simulink model "flc_ruido"  (R2023a)
settings: Solver=VariableStepAuto  StartTime=0.0  StopTime=1000  RelTol=1e-3
values from neighbouring files (symbols this model uses):
  A = 0.0154    [parametros.m]    (also in variables.mat)
  az1 = 1    [parametros.m]    (also in variables.mat)
  az2 = 1    [parametros.m]    (also in variables.mat)
  az3 = 1    [parametros.m]    (also in variables.mat)
  g = 9.8    [parametros.m]    (also in variables.mat)
  H_star1 = 0.4    [parametros.m]    (also in variables.mat)
  H_star2 = 0.15    [parametros.m]    (also in variables.mat)
  Sn = 5e-5    (= 5e-05)    [parametros.m]    (also in variables.mat)
libraries: fuzblock x2
settings Model: Creator=empg0  LastModifiedBy=empg0

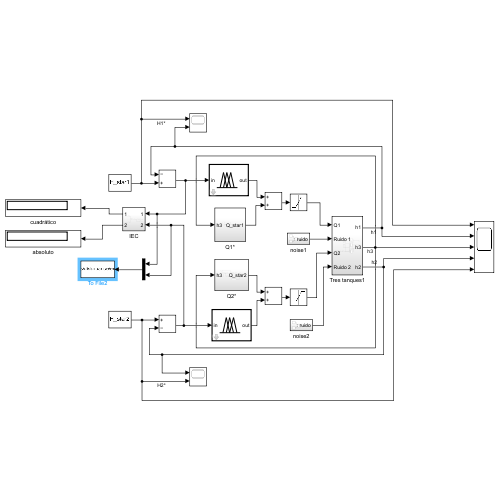
[thumbnail: Simulink's stored preview of the top-level diagram]
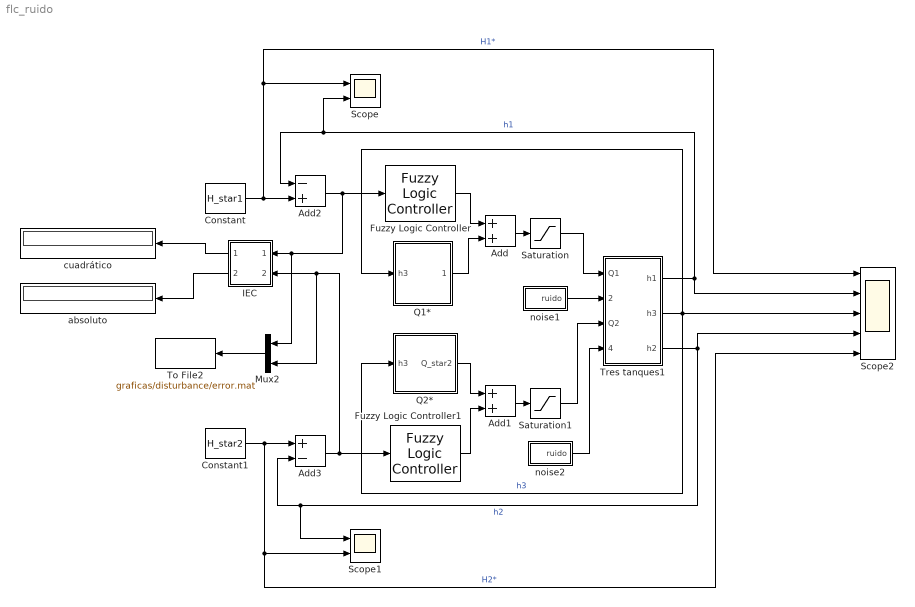
== system flc_ruido ==
  Add : Sum
  Add1 : Sum
  Add2 : Sum  Inputs=-+
  Add3 : Sum  Inputs=+-
  Constant : Constant  Value=H_star1
  Constant1 : Constant  Value=H_star2
  Fuzzy Logic Controller : fuzblock/Fuzzy Logic  Controller  FIS='error_fuzzy.fis'  OutputSampleNumber=101  DataType=double  FuzzifiedInputs=off  RuleFiringStrengths=off  RuleOutputs=off  AggregatedOutputs=off  SimulateUsing=Interpreted execution  OutOfRangeInputValueMessage=warning  NoRuleFiredMessage=warning  EmptyOutputFuzzySetMessage=warning
  Fuzzy Logic Controller1 : fuzblock/Fuzzy Logic  Controller  FIS='error_fuzzy.fis'  OutputSampleNumber=101  DataType=double  FuzzifiedInputs=off  RuleFiringStrengths=off  RuleOutputs=off  AggregatedOutputs=off  SimulateUsing=Interpreted execution  OutOfRangeInputValueMessage=warning  NoRuleFiredMessage=warning  EmptyOutputFuzzySetMessage=warning
  IEC : Subsystem
  Mux2 : Mux  Inputs=2
  Q1* : Subsystem
  Q2* : Subsystem
  Saturation : Saturate  UpperLimit=0.1  LowerLimit=0
  Saturation1 : Saturate  UpperLimit=0.1  LowerLimit=0
  Scope : Scope  NumInputPorts=2
  Scope1 : Scope  NumInputPorts=2
  Scope2 : Scope  NumInputPorts=5
  To File2 : ToFile  Filename=graficas/disturbance/error.mat  MatrixName=error  SampleTime=0.5
  Tres tanques1 : Subsystem
  absoluto : Display
  cuadrático : Display
  noise1 : Subsystem
  noise2 : Subsystem
  wires:
  Fuzzy Logic Controller/1 -> Add/1
  Q1*/1(Q_star1) -> Add/2
  Q2*/1(Q_star2) -> Add1/1
  Fuzzy Logic Controller1/1 -> Add1/2
  Constant/1 -> Scope/1, Scope2/1, Add2/2  "H1*"
  Add2/1 -> Mux2/1, IEC/1(In1), Fuzzy Logic Controller/1
  Tres tanques1/1(h1) -> Scope2/2, Scope/2, Add2/1  "h1"
  Add3/1 -> Mux2/2, IEC/2(In2), Fuzzy Logic Controller1/1
  Constant1/1 -> Scope1/2, Scope2/5, Add3/1  "H2*"
  Tres tanques1/3(h2) -> Scope2/4, Scope1/1, Add3/2  "h2"
  Tres tanques1/2(h3) -> Scope2/3, Q1*/1(h3), Q2*/1(h3)  "h3"
  Add/1 -> Saturation/1
  Add1/1 -> Saturation1/1
  IEC/1(Out1) -> cuadrático/1
  Mux2/1 -> To File2/1
  Saturation/1 -> Tres tanques1/1(Q1)
  Saturation1/1 -> Tres tanques1/3(Q2)
  noise1/1(ruido) -> Tres tanques1/2(Ruido 1)
  noise2/1(ruido) -> Tres tanques1/4(Ruido 2)
  IEC/2(Out2) -> absoluto/1

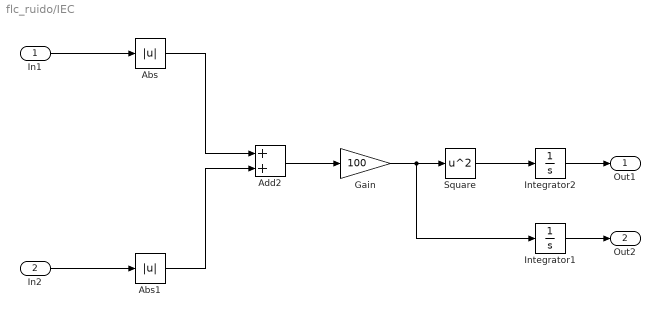
== system flc_ruido/IEC ==
  In1 : Inport
  In2 : Inport  Port=2
  Abs : Abs  SaturateOnIntegerOverflow=off
  Abs1 : Abs  SaturateOnIntegerOverflow=off
  Add2 : Sum
  Gain : Gain  Gain=100
  Integrator1 : Integrator
  Integrator2 : Integrator
  Square : Math  Operator=square
  Out1 : Outport
  Out2 : Outport  Port=2
  wires:
  Abs1/1 -> Add2/2
  Abs/1 -> Add2/1
  In2/1 -> Abs1/1
  Square/1 -> Integrator2/1
  Integrator2/1 -> Out1/1
  In1/1 -> Abs/1
  Add2/1 -> Gain/1
  Gain/1 -> Integrator1/1, Square/1
  Integrator1/1 -> Out2/1

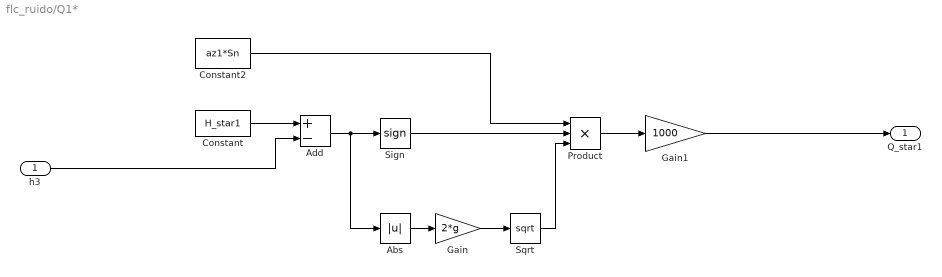
== system flc_ruido/Q1* ==
  h3 : Inport
  Abs : Abs  SaturateOnIntegerOverflow=off
  Add : Sum  Inputs=+-
  Constant : Constant  Value=H_star1
  Constant2 : Constant  Value=az1*Sn
  Gain : Gain  Gain=2*g
  Gain1 : Gain  Gain=1000
  Product : Product  Inputs=3
  Sign : Signum
  Sqrt : Sqrt
  Q_star1 : Outport
  wires:
  Product/1 -> Gain1/1
  Gain/1 -> Sqrt/1
  h3/1 -> Add/2
  Add/1 -> Abs/1, Sign/1
  Abs/1 -> Gain/1
  Constant/1 -> Add/1
  Sqrt/1 -> Product/3
  Constant2/1 -> Product/1
  Sign/1 -> Product/2
  Gain1/1 -> Q_star1/1

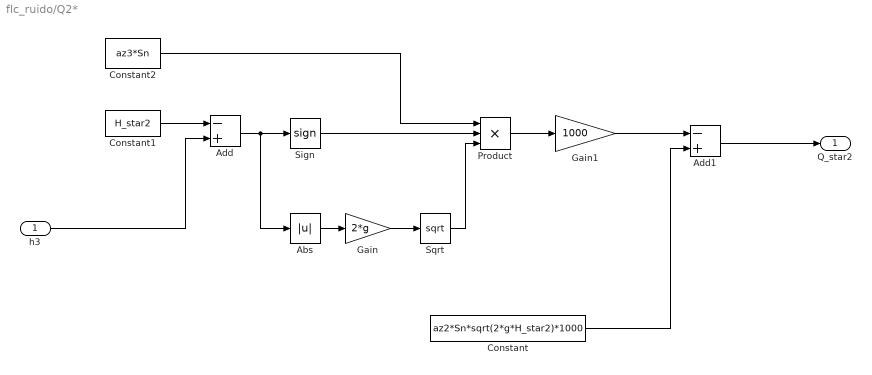
== system flc_ruido/Q2* ==
  h3 : Inport
  Abs : Abs  SaturateOnIntegerOverflow=off
  Add : Sum  Inputs=-+
  Add1 : Sum  Inputs=-+
  Constant : Constant  Value=az2*Sn*sqrt(2*g*H_star2)*1000
  Constant1 : Constant  Value=H_star2
  Constant2 : Constant  Value=az3*Sn
  Gain : Gain  Gain=2*g
  Gain1 : Gain  Gain=1000
  Product : Product  Inputs=3
  Sign : Signum
  Sqrt : Sqrt
  Q_star2 : Outport
  wires:
  Add1/1 -> Q_star2/1
  Sign/1 -> Product/2
  Sqrt/1 -> Product/3
  Product/1 -> Gain1/1
  Constant1/1 -> Add/1
  Add/1 -> Abs/1, Sign/1
  Abs/1 -> Gain/1
  Constant2/1 -> Product/1
  Gain/1 -> Sqrt/1
  Constant/1 -> Add1/2
  Gain1/1 -> Add1/1
  h3/1 -> Add/2

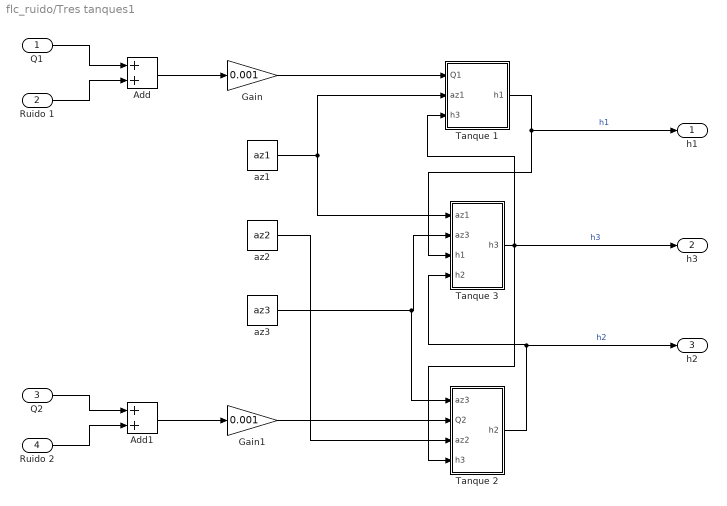
== system flc_ruido/Tres tanques1 ==
  Q1 : Inport
  Ruido 1 : Inport  Port=2
  Q2 : Inport  Port=3
  Ruido 2 : Inport  Port=4
  Add : Sum
  Add1 : Sum
  Gain : Gain  Gain=0.001
  Gain1 : Gain  Gain=0.001
  Tanque 1 : Subsystem
  Tanque 2 : Subsystem
  Tanque 3 : Subsystem
  az1 : Constant  Value=az1
  az2 : Constant  Value=az2
  az3 : Constant  Value=az3
  h1 : Outport
  h3 : Outport  Port=2
  h2 : Outport  Port=3
  wires:
  Tanque 2/1(h2) -> Tanque 3/4(h2), h2/1  "h2"
  Tanque 1/1(h1) -> Tanque 3/3(h1), h1/1  "h1"
  Gain1/1 -> Tanque 2/2(Q2)
  Tanque 3/1(h3) -> Tanque 2/4(h3), h3/1, Tanque 1/3(h3)  "h3"
  az3/1 -> Tanque 2/1(az3), Tanque 3/2(az3)
  az1/1 -> Tanque 3/1(az1), Tanque 1/2(az1)
  az2/1 -> Tanque 2/3(az2)
  Gain/1 -> Tanque 1/1(Q1)
  Add/1 -> Gain/1
  Q1/1 -> Add/1
  Ruido 1/1 -> Add/2
  Add1/1 -> Gain1/1
  Q2/1 -> Add1/1
  Ruido 2/1 -> Add1/2

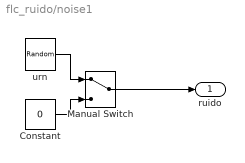
== system flc_ruido/noise1 ==
  Constant : Constant  Value=0
  Manual Switch : ManualSwitch
  urn : UniformRandomNumber  Minimum=-0.1*0.1  Maximum=0.1*0.1  Seed=140  SampleTime=20
  ruido : Outport
  wires:
  urn/1 -> Manual Switch/1
  Constant/1 -> Manual Switch/2
  Manual Switch/1 -> ruido/1

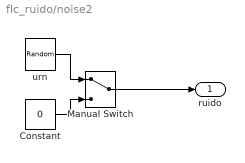
== system flc_ruido/noise2 ==
  Constant : Constant  Value=0
  Manual Switch : ManualSwitch
  urn : UniformRandomNumber  Minimum=-0.1*0.1  Maximum=0.1*0.1  Seed=150  SampleTime=20
  ruido : Outport
  wires:
  urn/1 -> Manual Switch/1
  Constant/1 -> Manual Switch/2
  Manual Switch/1 -> ruido/1

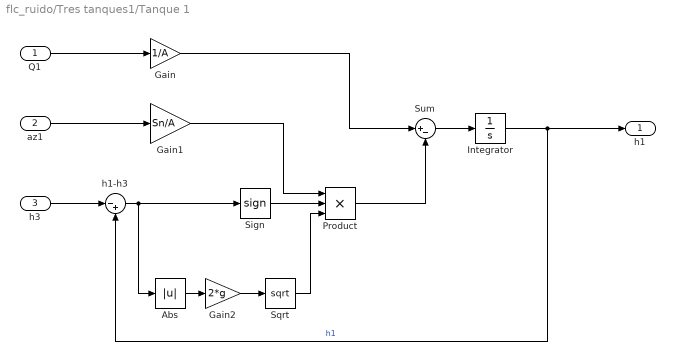
== system flc_ruido/Tres tanques1/Tanque 1 ==
  Q1 : Inport
  az1 : Inport  Port=2
  h3 : Inport  Port=3
  Abs : Abs  SaturateOnIntegerOverflow=off
  Gain : Gain  Gain=1/A
  Gain1 : Gain  Gain=Sn/A
  Gain2 : Gain  Gain=2*g
  Integrator : Integrator  LimitOutput=on  UpperSaturationLimit=0.62  LowerSaturationLimit=0
  Product : Product  Inputs=3
  Sign : Signum
  Sqrt : Sqrt
  Sum : Sum  Inputs=|+-
  h1-h3 : Sum  Inputs=|-+
  h1 : Outport
  wires:
  h3/1 -> h1-h3/1
  Sum/1 -> Integrator/1
  Gain2/1 -> Sqrt/1
  Gain1/1 -> Product/1
  Sqrt/1 -> Product/3
  Sign/1 -> Product/2
  h1-h3/1 -> Abs/1, Sign/1
  Q1/1 -> Gain/1
  az1/1 -> Gain1/1
  Integrator/1 -> h1/1, h1-h3/2  "h1"
  Product/1 -> Sum/2
  Gain/1 -> Sum/1
  Abs/1 -> Gain2/1

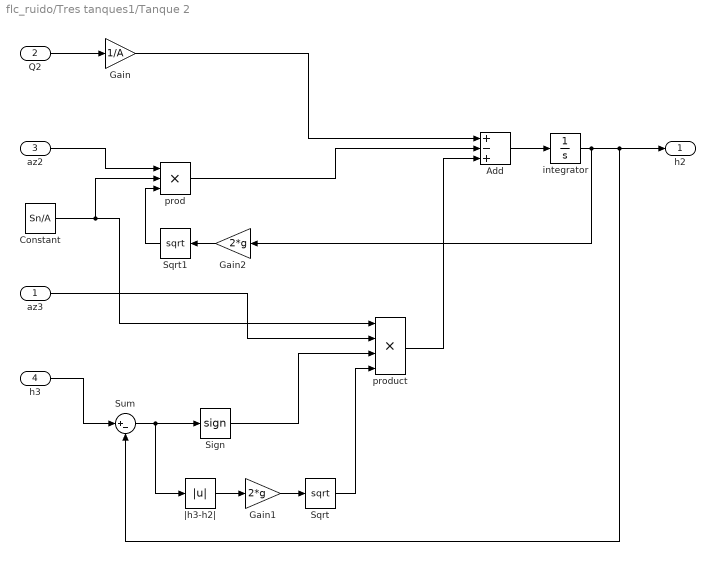
== system flc_ruido/Tres tanques1/Tanque 2 ==
  az3 : Inport
  Q2 : Inport  Port=2
  az2 : Inport  Port=3
  h3 : Inport  Port=4
  Add : Sum  Inputs=+-+
  Constant : Constant  Value=Sn/A
  Gain : Gain  Gain=1/A
  Gain1 : Gain  Gain=2*g
  Gain2 : Gain  Gain=2*g
  Sign : Signum
  Sqrt : Sqrt
  Sqrt1 : Sqrt
  Sum : Sum  Inputs=|+-
  integrator : Integrator  LimitOutput=on  UpperSaturationLimit=0.62  LowerSaturationLimit=0
  prod : Product  Inputs=3
  product : Product  Inputs=4
  |h3-h2| : Abs  SaturateOnIntegerOverflow=off
  h2 : Outport
  wires:
  |h3-h2|/1 -> Gain1/1
  prod/1 -> Add/2
  product/1 -> Add/3
  Add/1 -> integrator/1
  Gain/1 -> Add/1
  Constant/1 -> product/1, prod/2
  Gain1/1 -> Sqrt/1
  Sum/1 -> |h3-h2|/1, Sign/1
  az2/1 -> prod/1
  az3/1 -> product/2
  Sqrt1/1 -> prod/3
  Sqrt/1 -> product/4
  Sign/1 -> product/3
  h3/1 -> Sum/1
  integrator/1 -> Gain2/1, h2/1, Sum/2
  Gain2/1 -> Sqrt1/1
  Q2/1 -> Gain/1

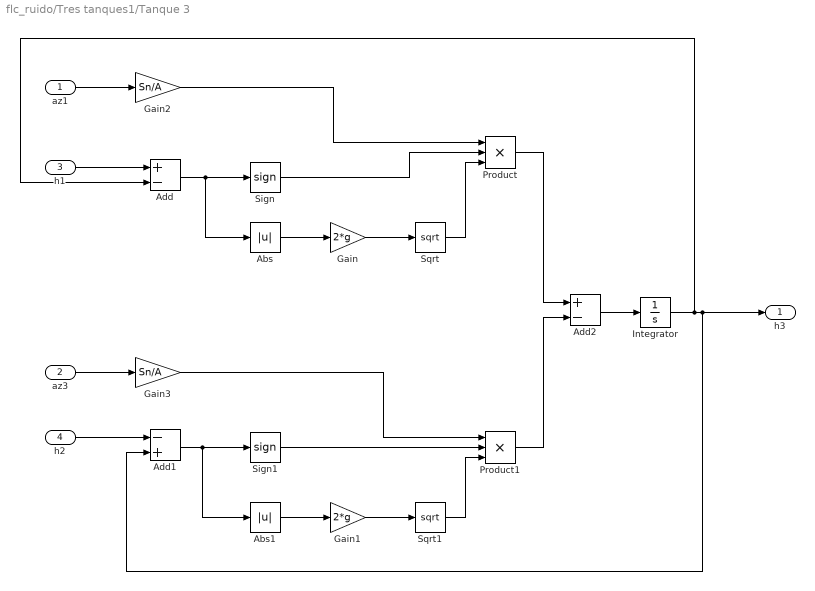
== system flc_ruido/Tres tanques1/Tanque 3 ==
  az1 : Inport
  az3 : Inport  Port=2
  h1 : Inport  Port=3
  h2 : Inport  Port=4
  Abs : Abs  SaturateOnIntegerOverflow=off
  Abs1 : Abs  SaturateOnIntegerOverflow=off
  Add : Sum  Inputs=+-
  Add1 : Sum  Inputs=-+
  Add2 : Sum  Inputs=+-
  Gain : Gain  Gain=2*g
  Gain1 : Gain  Gain=2*g
  Gain2 : Gain  Gain=Sn/A
  Gain3 : Gain  Gain=Sn/A
  Integrator : Integrator  LimitOutput=on  UpperSaturationLimit=0.62  LowerSaturationLimit=0
  Product : Product  Inputs=3
  Product1 : Product  Inputs=3
  Sign : Signum
  Sign1 : Signum
  Sqrt : Sqrt
  Sqrt1 : Sqrt
  h3 : Outport
  wires:
  Add2/1 -> Integrator/1
  Gain3/1 -> Product1/1
  az1/1 -> Gain2/1
  Gain1/1 -> Sqrt1/1
  Add1/1 -> Abs1/1, Sign1/1
  h1/1 -> Add/1
  az3/1 -> Gain3/1
  Integrator/1 -> h3/1, Add1/2, Add/2
  Abs1/1 -> Gain1/1
  Add/1 -> Abs/1, Sign/1
  Abs/1 -> Gain/1
  Sqrt1/1 -> Product1/3
  Sign/1 -> Product/2
  Product1/1 -> Add2/2
  Gain2/1 -> Product/1
  Sqrt/1 -> Product/3
  Sign1/1 -> Product1/2
  Gain/1 -> Sqrt/1
  h2/1 -> Add1/1
  Product/1 -> Add2/1
